simulink library "SUB_ECU_L4_MABX_HW_Interface"  (R2018a)
settings: Solver=VariableStepAuto  StartTime=0.0  StopTime=10.0  RelTol=1e-3
PostLoadFcn:
  | , if any(exist('dsrtsu_mdlpostloadfcn', 'file') == [2, 3, 6]), try dsrtsu_mdlpostloadfcn('Execute', bdroot); catch fprintf('Error in PostLoadFcn (dsrtsu_mdlpostloadfcn) for model "%s":\n %s\n', bdroot, lasterr); end, end,
undefined symbols (not defined in the file or in its folder): CANR_PROPB_REAX_3_13_CHANNEL_APV, CANR_PROPB_REAX_4_13_CHANNEL_APV, CANR_PROPB_XPR_1_50_CHANNEL_APV, ENUM_CAN_RX_T, ENUM_CAN_TX_T, ENUM_REAX_OPERATION_MODE_T, ENUM_SIGNAL_HEALTH_T, ENUM_XBR_CONTROL_MODE_T, ENUM_XBR_EBI_MODE_T, ENUM_XBR_PASS_THROUGH_ACTIVE_T, ENUM_XBR_PRIORITY_T, ENUM_XPR_INHIBIT_PARK_MANUAL_T, ENUM_XPR_INHIBIT_UNPARK_MANUAL_T, ENUM_XPR_PARK_MANUAL_T, ENUM_XPR_UNPARK_MANUAL_T, PROPB_REAX_1_E4_DES_POS_SIG_SRC_APV, PROPB_REAX_1_E4_DESIRED_OPMODE_APV, PROPB_REAX_1_E4_DESIRED_POSITION_APV, ptc_matlab_lib
libraries: PTC_MBDS_LIB x264, rtican x172, EmE_MBD_Blockset x39, simulink x34, $bdroot x16, rti1401lib_dio_type4 x8, simulink_need_slupdate x7, dsa_tcpip_lib x4, rti1401lib_adc_type4 x3, rtmapslib x3, rtitasklib x3
(part 14 of 51)

== system SUB_ECU_L4_MABX_HW_Interface/CAN_PIC_KW/CAN_RX_CCVS1_31/RX_CAN_31 ==
  Enable : Inport
  Bus Creator : BusCreator  Inputs=20
  Bus Creator3 : BusCreator  Inputs=4
  CCVS1_31 : rtican/RTICAN Receive (RX)   Reserved1=[]  Reserved2=[]  Reserved3=[]  Reserved4=[]  SfcnMessage=[]  Msg_Struct=[]  BoardTypeNo=[]  BoardNo=[]  ChannelNo=[]  Parameters=[]  DialogFcn=[]  UnitName=[]  Revision=[]  UnitValues=[]  DSProperties=struct('RTI',struct('Version',uint32(5),'BlockType',struct('isSLSource',uint8(1),'isSLSink',uint8(1),'isHWSource',uint8(0),'isHWSink',uint8(0),'isSetup',uint8(0),'isInline',uint8(1),'isNonInline',uint8(0),'isInterrupt',uint8(0),'isChannelwise',uint8(0)),'IOBoardType','RTICAN','UnitType','MESSAGE','Identifier','RX','DialogType','MSVC','BlockSet','RTICAN','SlaveProcessor','CAN'))  RTIBlockInterface=struct('OutputPortsWidth',int32([1 1 1 1 1 1 1 1 1 1 1 1 1 1 1 1 1 1 1 1 1 1 1]),'OutputPortsActive',ones(1,23),'OutputPortsName',{{'TwoSpeedAxleSwitch','ParkingBrakeSwitch','CruiseCtrlPauseSwitch','ParkBrakeReleaseInhibitRq','WheelBasedVehicleSpeed','CruiseCtrlActive','CruiseCtrlEnableSwitch','BrakeSwitch','ClutchSwitch','CruiseCtrlSetSwitch','CruiseCtrlCoastSwitch','CruiseCtrlResumeSwitch','CruiseCtrlAccelerateSwitch','CruiseCtrlSetSpeed','PTOGovernorState','CruiseCtrlStates','EngIdleIncrementSwitch','EngIdleDecrementSwitch','EngTestModeSwitch','EngShutdownOverrideSwitch',['RX status'],['RX time'],['RX delta time']}},'OutputPortsDataType',{{'SS_DOUBLE','SS_DOUBLE','SS_DOUBLE','SS_DOUBLE','SS_DOUBLE','SS_DOUBLE','SS_DOUBLE','SS_DOUBLE','SS_DOUBLE','SS_DOUBLE','SS_DOUBLE','SS_DOUBLE','SS_DOUBLE','SS_DOUBLE','SS_DOUBLE','SS_DOUBLE','SS_DOUBLE','SS_DOUBLE','SS_DOUBLE','SS_DOUBLE','SS_DOUBLE','SS_DOUBLE','SS_DOUBLE'}},'OutputPortsLabel',{{'TwoSpeedAxleSwitch','ParkingBrakeSwitch','CruiseCtrlPauseSwitch','ParkBrakeReleaseInhibitRq','WheelBasedVehicleSpeed','CruiseCtrlActive','CruiseCtrlEnableSwitch','BrakeSwitch','ClutchSwitch','CruiseCtrlSetSwitch','CruiseCtrlCoastSwitch','CruiseCtrlResumeSwitch','CruiseCtrlAccelerateSwitch','CruiseCtrlSetSpeed','PTOGovernorState','CruiseCtrlStates','EngIdleIncrementSwitch','EngIdleDecrementSwitch','EngTestModeSwitch','EngShutdownOverrideSwitch','','',''}},'OutputPortsLabelMode','ON','InputPortsWidth',int32(0),'InputPortsActive',0,'DialogFcn','rtican_message_interface_gui','BlockDisplay',{{'','center'}},'IconTransparency','on','ParameterTunableNames',{{}},'InitLevel',3,'BlockName',struct('Token',{{'CCVS1_31'}}),'SampleTime',{{-1}},'TriggerPort',{{'none'}},'EnablePort',{{'yes'}})  RTIBlockParameters=struct('BoardTypeNo',{{1,'OFF',[]}},'BoardNo',{{1,'ON',[1 16]}},'ChannelNo',{{1,'ON',[1 2]}},'Parameters',{{struct('DataFileSupport',struct('DataFileSelectedMaster',1,'DataFileSelectedLocal',0,'DataFileName','c:\localdata\chris\advanced_tech\adas\level4_rcp\truck1571\dbc\mabx_can1.dbc|','DataFileDate',{{{['03-Apr-2017 12:55:40']}}},'SelectedFile',['<no file selected>']),'Options',struct('StatusSelected',1,'TimeSelected',1,'DeltaTimeSelected',1,'BytePortSelected',0,'MessageLengthSelected',0,'TriggerPort',struct('Selected',0,'TriggerType',0),'UserCoding',struct('Selected',0,'InterfaceFile','UserDecodingFile','FcnName','UserDecodeFcn','InportSelected',0,'InportWidth',1,'OutportSelected',0,'OutportWidth',1),'EnablePortSelected',1,'SignalOnPortnameSelected',1,'UseRXService',1),'Message',struct('MsgOnBlocknameSelected',1,'MsgName','CCVS1_31','MsgIdFormat',1,'MsgId',419361073,'MsgLength',8,'NumSignals',20,'SampleTime',-1,'Signal',struct('SgnName',{'TwoSpeedAxleSwitch','ParkingBrakeSwitch','CruiseCtrlPauseSwitch','ParkBrakeReleaseInhibitRq','WheelBasedVehicleSpeed','CruiseCtrlActive','CruiseCtrlEnableSwitch','BrakeSwitch','ClutchSwitch','CruiseCtrlSetSwitch','CruiseCtrlCoastSwitch','CruiseCtrlResumeSwitch','CruiseCtrlAccelerateSwitch','CruiseCtrlSetSpeed','PTOGovernorState','CruiseCtrlStates','EngIdleIncrementSwitch','EngIdleDecrementSwitch','EngTestModeSwitch','EngShutdownOverrideSwitch'},'SgnStartBit',{0,2,4,6,8,24,26,28,30,32,34,36,38,40,48,53,56,58,60,62},'SgnLength',{2,2,2,2,16,2,2,2,2,2,2,2,2,8,5,3,2,2,2,2},'SgnType',{0,0,0,0,0,0,0,0,0,0,0,0,0,0,0,0,0,0,0,0},'ModeValue',{-1,-1,-1,-1,-1,-1,-1,-1,-1,-1,-1,-1,-1,-1,-1,-1,-1,-1,-1,-1},'DataType',{0,0,0,0,0,0,0,0,0,0,0,0,0,0,0,0,0,0,0,0},'ByteLayout',{0,0,0,0,0,0,0,0,0,0,0,0,0,0,0,0,0,0,0,0},'Factor',{1,1,1,1,2^-8,1,1,1,1,1,1,1,1,1,1,1,1,1,1,1},'Offset',{0,0,0,0,0,0,0,0,0,0,0,0,0,0,0,0,0,0,0,0},'SgnComment',{{['Switch signal which indicates the current axle range.']},{['Switch signal which indicates when the parking brake is set.']},{['Switch signal which indicates the position of the Cruise Control Pause Switch used on Remote Cruise Control applications.']},{['Park Brake Release Inhibit Request signals the desire that an applied park brake remain applied and limit the ability of the']},{['Speed of the vehicle as calculated from wheel or tailshaft speed.']},{['Cruise control is switched on.']},{['Switch signal which indicates that it is possible to manage the cruise control function.']},{['Switch signal which indicates that the driver operated brake foot pedal is being pressed.']},{['Switch signal which indicates that the clutch pedal is being pressed.']},{['Switch signal of the cruise control activator which indicates that the activator is in the position “set.']},{['Switch signal of the cruise control activator which indicates that the activator is in the position “coast (decelerate).']},{['Switch signal of the cruise control activator which indicates that the activator is in the position “resume.']},{['Switch signal of the cruise control activator which indicates that the activator is in the position “accelerate.']},{['Value of set (chosen) velocity of velocity control system.']},{['This parameter is used to indicate the current state or mode of operation by the power takeoff (PTO) governor.']},{['This parameter is used to indicate the current state, or mode, of operation by the cruise control device.']},{['Switch signal which indicates the position of the idle increment switch.']},{['Switch signal which indicates the position of the idle decrement switch.']},{['Switch signal which indicates the position of the engine test mode switch.']},{['Switch signal which indicates the position of the engine shutdown override switch.']}},'SgnUnit',{'','','','','km/h','','','','','','','','','km/h','','','','','',''},'Min',{0,0,0,0,0,0,0,0,0,0,0,0,0,0,0,0,0,0,0,0},'Max',{3,3,3,3,250.996,3,3,3,3,3,3,3,3,250,31,7,3,3,3,3},'SLDataType',{'SS_DOUBLE','SS_DOUBLE','SS_DOUBLE','SS_DOUBLE','SS_DOUBLE','SS_DOUBLE','SS_DOUBLE','SS_DOUBLE','SS_DOUBLE','SS_DOUBLE','SS_DOUBLE','SS_DOUBLE','SS_DOUBLE','SS_DOUBLE','SS_DOUBLE','SS_DOUBLE','SS_DOUBLE','SS_DOUBLE','SS_DOUBLE','SS_DOUBLE'}),'MsgIdNumFormat',1,'MsgComment',{{['Cruise Control/Vehicle Speed']}}),'Version',1.2,'general',struct('isFromLib',0)),'OFF',[]}},'GroupId',{{struct('Group',{{'RTICAN'}},'No',25,'Behavior',{{'NAMECHANGE'}},'BlockType',{{'SINK'}},'NameChangeFlag',0),'OFF',[]}},'SFcnRTICANMessage',{{struct('MsgType','RX','SFcnPortType','Scalar','MsgName','CCVS1_31','MsgIdFormat','XTD','MsgId',419361073,'MsgLength',8,'NumSignals',20,'SampleTime',-1,'Signal',struct('SgnName',{'TwoSpeedAxleSwitch','ParkingBrakeSwitch','CruiseCtrlPauseSwitch','ParkBrakeReleaseInhibitRq','WheelBasedVehicleSpeed','CruiseCtrlActive','CruiseCtrlEnableSwitch','BrakeSwitch','ClutchSwitch','CruiseCtrlSetSwitch','CruiseCtrlCoastSwitch','CruiseCtrlResumeSwitch','CruiseCtrlAccelerateSwitch','CruiseCtrlSetSpeed','PTOGovernorState','CruiseCtrlStates','EngIdleIncrementSwitch','EngIdleDecrementSwitch','EngTestModeSwitch','EngShutdownOverrideSwitch'},'SgnStartBit',{0,2,4,6,8,24,26,28,30,32,34,36,38,40,48,53,56,58,60,62},'SgnLength',{2,2,2,2,16,2,2,2,2,2,2,2,2,8,5,3,2,2,2,2},'SgnType',{'standard','standard','standard','standard','standard','standard','standard','standard','standard','standard','standard','standard','standard','standard','standard','standard','standard','standard','standard','standard'},'ModeValue',{-1,-1,-1,-1,-1,-1,-1,-1,-1,-1,-1,-1,-1,-1,-1,-1,-1,-1,-1,-1},'DataType',{['unsigned int'],['unsigned int'],['unsigned int'],['unsigned int'],['unsigned int'],['unsigned int'],['unsigned int'],['unsigned int'],['unsigned int'],['unsigned int'],['unsigned int'],['unsigned int'],['unsigned int'],['unsigned int'],['unsigned int'],['unsigned int'],['unsigned int'],['unsigned int'],['unsigned int'],['unsigned int']},'ByteLayout',{['little endian'],['little endian'],['little endian'],['little endian'],['little endian'],['little endian'],['little endian'],['little endian'],['little endian'],['little endian'],['little endian'],['little endian'],['little endian'],['little endian'],['little endian'],['little endian'],['little endian'],['little endian'],['little endian'],['little endian']},'Factor',{1,1,1,1,2^-8,1,1,1,1,1,1,1,1,1,1,1,1,1,1,1},'Offset',{0,0,0,0,0,0,0,0,0,0,0,0,0,0,0,0,0,0,0,0},'SLDataType',{'SS_DOUBLE','SS_DOUBLE','SS_DOUBLE','SS_DOUBLE','SS_DOUBLE','SS_DOUBLE','SS_DOUBLE','SS_DOUBLE','SS_DOUBLE','SS_DOUBLE','SS_DOUBLE','SS_DOUBLE','SS_DOUBLE','SS_DOUBLE','SS_DOUBLE','SS_DOUBLE','SS_DOUBLE','SS_DOUBLE','SS_DOUBLE','SS_DOUBLE'}),'StatusSelected','yes','TimeSelected','yes','DeltaTimeSelected','yes','BytePortSelected','no','MessageLengthSelected','no','TriggerPort',struct('Selected','no','TriggerType',0),'UserCoding',struct('Selected','no','InterfaceFile','UserDecodingFile','FcnName','UserDecodeFcn','InportSelected','no','InportWidth',1,'OutportSelected','no','OutportWidth',1),'EnablePortSelected','yes','UseRXService','yes','BoardType','DS1','BoardNo',1,'ControllerNo',1),'OFF',[]}},'TLCFileName',{{'rtican_rx_message','OFF',[]}})  RTISFcnParameters=struct('SFcnRTICANMessage','struct','TLCFileName','char')  RTIBlockParaDefault=struct('BoardTypeNo',4302,'BoardNo',1,'ChannelNo',1,'Parameters',struct('DataFileSupport',struct('DataFileSelectedMaster',0,'DataFileSelectedLocal',0,'DataFileName','','DataFileDate','','SelectedFile',['<no file selected>']),'Options',struct('StatusSelected',1,'TimeSelected',1,'DeltaTimeSelected',1,'BytePortSelected',0,'MessageLengthSelected',0,'TriggerPort',struct('Selected',0,'TriggerType','rising'),'UserCoding',struct('Selected',0,'InterfaceFile','UserDecodingFile','FcnName','UserDecodeFcn','InportSelected',0,'InportWidth',1,'OutportSelected',0,'OutportWidth',1),'EnablePortSelected',0,'SignalOnPortnameSelected',1,'UseRXService',0),'Message',struct('MsgOnBlocknameSelected',0,'MsgName',['RX Message'],'MsgIdFormat',0,'MsgId',100,'MsgLength',8,'NumSignals',1,'SampleTime',-1,'Signal',struct('SgnName',['RX signal'],'SgnStartBit',0,'SgnLength',8,'SgnType',0,'ModeValue',-1,'DataType',0,'SLDataType','SS_DOUBLE','ByteLayout',0,'Factor',1,'Offset',0,'Min',0,'Max',255,'SgnComment',{{}},'SgnUnit',''),'MsgIdNumFormat',0,'MsgComment',{{''}}),'Version',1.2,'general',struct('isFromLib',1)),'GroupId',struct('Group',{{'RTICAN'}},'No',1,'Behavior',{{'NAMECHANGE'}},'BlockType',{{'SINK'}},'NameChangeFlag',0),'SFcnRTICANMessage',struct('MsgType','RX','MsgName',['RX Message'],'MsgIdFormat','STD','MsgId',100,'MsgLength',8,'NumSignals',1,'SampleTime',-1,'Signal',struct('SgnName',['RX signal'],'SgnStartBit',0,'SgnLength',8,'SgnType','standard','ModeValue',-1,'DataType',['unsigned int'],'ByteLayout',['little endian'],'SLDataType','SS_DOUBLE','Factor',1,'Offset',0),'StatusSelected','yes','TimeSelected','yes','DeltaTimeSelected','yes','BytePortSelected','no','MessageLengthSelected','no','EnablePortSelected','no','UserCoding',struct('Selected','no','InterfaceFile','UserDecodingFile','FcnName','UserDecodeFcn','InportSelected','no','InportWidth',1,'OutportSelected','no','OutportWidth',1),'TriggerPort',struct('Selected','no','TriggerType','rising'),'UseRXService','no','BoardType','DS4302','BoardNo',1,'ControllerNo',1,'SFcnPortType','Scalar'),'TLCFileName','rtican_rx_message')
      settings: AttributesFormatString=Group Id: RTICAN25\n  SourceProductName=dSPACE RTI CAN Blockset
  Data Type Conversion10 : DataTypeConversion  OutDataTypeStr=double  SaturateOnIntegerOverflow=on
  Data Type Conversion8 : DataTypeConversion  OutDataTypeStr=boolean  SaturateOnIntegerOverflow=on
  Data Type Conversion9 : DataTypeConversion  OutDataTypeStr=double  SaturateOnIntegerOverflow=on
  CCVS1_31_ : Outport
  wires:
  Bus Creator3/1 -> CCVS1_31_/1  "CCVS1_31"
  Bus Creator/1 -> Bus Creator3/1  "CCVS31Data"
  Enable/1 -> CCVS1_31/Enable
  CCVS1_31/23 -> Data Type Conversion10/1
  CCVS1_31/22 -> Data Type Conversion9/1
  CCVS1_31/21 -> Data Type Conversion8/1
  Data Type Conversion8/1 -> Bus Creator3/2  "RX_status"
  Data Type Conversion10/1 -> Bus Creator3/4  "RX_delta_time"
  Data Type Conversion9/1 -> Bus Creator3/3  "RX_time"
  CCVS1_31/13 -> Bus Creator/13  "CruiseCtrlAccelerateSwitch"
  CCVS1_31/12 -> Bus Creator/12  "CruiseCtrlResumeSwitch"
  CCVS1_31/11 -> Bus Creator/11  "CruiseCtrlCoastSwitch"
  CCVS1_31/16 -> Bus Creator/16  "CruiseCtrlStates"
  CCVS1_31/14 -> Bus Creator/14  "CruiseCtrlSetSpeed"
  CCVS1_31/15 -> Bus Creator/15  "PTOGovernorState"
  CCVS1_31/8 -> Bus Creator/8  "BrakeSwitch"
  CCVS1_31/9 -> Bus Creator/9  "ClutchSwitch"
  CCVS1_31/10 -> Bus Creator/10  "CruiseCtrlSetSwitch"
  CCVS1_31/7 -> Bus Creator/7  "CruiseCtrlEnableSwitch"
  CCVS1_31/20 -> Bus Creator/20  "EngShutdownOverrideSwitch"
  CCVS1_31/19 -> Bus Creator/19  "EngTestModeSwitch"
  CCVS1_31/18 -> Bus Creator/18  "EngIdleDecrementSwitch"
  CCVS1_31/17 -> Bus Creator/17  "EngIdleIncrementSwitch"
  CCVS1_31/2 -> Bus Creator/2  "ParkingBrakeSwitch"
  CCVS1_31/1 -> Bus Creator/1  "TwoSpeedAxleSwitch"
  CCVS1_31/3 -> Bus Creator/3  "CruiseCtrlPauseSwitch"
  CCVS1_31/4 -> Bus Creator/4  "ParkBrakeReleaseInhibitRq"
  CCVS1_31/6 -> Bus Creator/6  "CruiseCtrlActive"
  CCVS1_31/5 -> Bus Creator/5  "WheelBasedVehicleSpeed"

== system SUB_ECU_L4_MABX_HW_Interface/CAN_PIC_KW/CAN_RX_COGSOGRapidUpdate_01/RX_CAN_4 ==
  Enable : Inport
  Bus Creator1 : BusCreator  Inputs=7
  Bus Creator3 : BusCreator  Inputs=7
  COGSOGRapidUpdate_00 : rtican/RTICAN Receive (RX)   Reserved1=[]  Reserved2=[]  Reserved3=[]  Reserved4=[]  SfcnMessage=[]  Msg_Struct=[]  BoardTypeNo=[]  BoardNo=[]  ChannelNo=[]  Parameters=[]  DialogFcn=[]  UnitName=[]  Revision=[]  UnitValues=[]  DSProperties=struct('RTI',struct('Version',uint32(5),'BlockType',struct('isSLSource',uint8(1),'isSLSink',uint8(1),'isHWSource',uint8(0),'isHWSink',uint8(0),'isSetup',uint8(0),'isInline',uint8(1),'isNonInline',uint8(0),'isInterrupt',uint8(0),'isChannelwise',uint8(0)),'IOBoardType','RTICAN','UnitType','MESSAGE','Identifier','RX','DialogType','MSVC','BlockSet','RTICAN','SlaveProcessor','CAN'))  RTIBlockInterface=struct('OutputPortsWidth',int32([1 1 1 1 1 1 1]),'OutputPortsActive',[1 1 1 1 1 1 1],'OutputPortsName',{{'SID','COGReference','CourseOverGround','SpeedOverGround',['RX status'],['RX time'],['RX delta time']}},'OutputPortsDataType',{{'SS_DOUBLE','SS_DOUBLE','SS_DOUBLE','SS_DOUBLE','SS_DOUBLE','SS_DOUBLE','SS_DOUBLE'}},'OutputPortsLabel',{{'SID','COGReference','CourseOverGround','SpeedOverGround','','',''}},'OutputPortsLabelMode','ON','InputPortsWidth',int32(0),'InputPortsActive',0,'DialogFcn','rtican_message_interface_gui','BlockDisplay',{{'','center'}},'IconTransparency','on','ParameterTunableNames',{{}},'InitLevel',3,'BlockName',struct('Token',{{'COGSOGRapidUpdate_00'}}),'SampleTime',{{-1}},'TriggerPort',{{'none'}},'EnablePort',{{'yes'}})  RTIBlockParameters=struct('BoardTypeNo',{{1,'OFF',[]}},'BoardNo',{{2,'ON',[1 16]}},'ChannelNo',{{2,'ON',[1 2]}},'Parameters',{{struct('DataFileSupport',struct('DataFileSelectedMaster',1,'DataFileSelectedLocal',0,'DataFileName','c:\localdata\chris\advanced_tech\adas\level4_rcp\truck1571\dbc\mabx_can4.dbc|','DataFileDate',{{{['10-Feb-2017 15:17:28']}}},'SelectedFile',['<no file selected>']),'Options',struct('StatusSelected',1,'TimeSelected',1,'DeltaTimeSelected',1,'BytePortSelected',0,'MessageLengthSelected',0,'TriggerPort',struct('Selected',0,'TriggerType',0),'UserCoding',struct('Selected',0,'InterfaceFile','UserDecodingFile','FcnName','UserDecodeFcn','InportSelected',0,'InportWidth',1,'OutportSelected',0,'OutportWidth',1),'EnablePortSelected',1,'SignalOnPortnameSelected',1,'UseRXService',1),'Message',struct('MsgOnBlocknameSelected',1,'MsgName','COGSOGRapidUpdate_00','MsgIdFormat',1,'MsgId',167248384,'MsgLength',8,'NumSignals',4,'SampleTime',-1,'Signal',struct('SgnName',{'SID','COGReference','CourseOverGround','SpeedOverGround'},'SgnStartBit',{0,8,16,32},'SgnLength',{8,2,16,16},'SgnType',{0,0,0,0},'ModeValue',{-1,-1,-1,-1},'DataType',{0,0,0,0},'ByteLayout',{0,0,0,0},'Factor',{1,1,0.0001,0.01},'Offset',{0,0,0,0},'SgnComment',{{['An upward counting number used to tie related information together between different PGNs.For example,SID would be used to tie together COG,SOG and RAIM values to a given Pos.255=no valid Pos fix to tie it to.Range 0 to 250 for valid Pos fixes.']},{['0 = True, ' char(10) '1 = Magnetic, ' char(10) '2 = Error, ' char(10) '3 = Null']},{['The direction of the path over ground actually followed by a vessel.']},{''}},'SgnUnit',{'','','rad','m/s'},'Min',{0,0,0,0},'Max',{252,3,6.28318,655.32},'SLDataType',{'SS_DOUBLE','SS_DOUBLE','SS_DOUBLE','SS_DOUBLE'}),'MsgIdNumFormat',1,'MsgComment',{{['This PGN is a single frame PGN that provides Course Over Ground(COG)and Speed Over Ground(SOG).' char(10) '' char(10) 'Being a ']}}),'Version',1.2,'general',struct('isFromLib',0)),'OFF',[]}},'GroupId',{{struct('Group',{{'RTICAN'}},'No',28,'Behavior',{{'NAMECHANGE'}},'BlockType',{{'SINK'}},'NameChangeFlag',0),'OFF',[]}},'SFcnRTICANMessage',{{struct('MsgType','RX','SFcnPortType','Scalar','MsgName','COGSOGRapidUpdate_00','MsgIdFormat','XTD','MsgId',167248384,'MsgLength',8,'NumSignals',4,'SampleTime',-1,'Signal',struct('SgnName',{'SID','COGReference','CourseOverGround','SpeedOverGround'},'SgnStartBit',{0,8,16,32},'SgnLength',{8,2,16,16},'SgnType',{'standard','standard','standard','standard'},'ModeValue',{-1,-1,-1,-1},'DataType',{['unsigned int'],['unsigned int'],['unsigned int'],['unsigned int']},'ByteLayout',{['little endian'],['little endian'],['little endian'],['little endian']},'Factor',{1,1,0.0001,0.01},'Offset',{0,0,0,0},'SLDataType',{'SS_DOUBLE','SS_DOUBLE','SS_DOUBLE','SS_DOUBLE'}),'StatusSelected','yes','TimeSelected','yes','DeltaTimeSelected','yes','BytePortSelected','no','MessageLengthSelected','no','TriggerPort',struct('Selected','no','TriggerType',0),'UserCoding',struct('Selected','no','InterfaceFile','UserDecodingFile','FcnName','UserDecodeFcn','InportSelected','no','InportWidth',1,'OutportSelected','no','OutportWidth',1),'EnablePortSelected','yes','UseRXService','yes','BoardType','DS1','BoardNo',2,'ControllerNo',2),'OFF',[]}},'TLCFileName',{{'rtican_rx_message','OFF',[]}})  RTISFcnParameters=struct('SFcnRTICANMessage','struct','TLCFileName','char')  RTIBlockParaDefault=struct('BoardTypeNo',4302,'BoardNo',1,'ChannelNo',1,'Parameters',struct('DataFileSupport',struct('DataFileSelectedMaster',0,'DataFileSelectedLocal',0,'DataFileName','','DataFileDate','','SelectedFile',['<no file selected>']),'Options',struct('StatusSelected',1,'TimeSelected',1,'DeltaTimeSelected',1,'BytePortSelected',0,'MessageLengthSelected',0,'TriggerPort',struct('Selected',0,'TriggerType','rising'),'UserCoding',struct('Selected',0,'InterfaceFile','UserDecodingFile','FcnName','UserDecodeFcn','InportSelected',0,'InportWidth',1,'OutportSelected',0,'OutportWidth',1),'EnablePortSelected',0,'SignalOnPortnameSelected',1,'UseRXService',0),'Message',struct('MsgOnBlocknameSelected',0,'MsgName',['RX Message'],'MsgIdFormat',0,'MsgId',100,'MsgLength',8,'NumSignals',1,'SampleTime',-1,'Signal',struct('SgnName',['RX signal'],'SgnStartBit',0,'SgnLength',8,'SgnType',0,'ModeValue',-1,'DataType',0,'SLDataType','SS_DOUBLE','ByteLayout',0,'Factor',1,'Offset',0,'Min',0,'Max',255,'SgnComment',{{}},'SgnUnit',''),'MsgIdNumFormat',0,'MsgComment',{{''}}),'Version',1.2,'general',struct('isFromLib',1)),'GroupId',struct('Group',{{'RTICAN'}},'No',1,'Behavior',{{'NAMECHANGE'}},'BlockType',{{'SINK'}},'NameChangeFlag',0),'SFcnRTICANMessage',struct('MsgType','RX','MsgName',['RX Message'],'MsgIdFormat','STD','MsgId',100,'MsgLength',8,'NumSignals',1,'SampleTime',-1,'Signal',struct('SgnName',['RX signal'],'SgnStartBit',0,'SgnLength',8,'SgnType','standard','ModeValue',-1,'DataType',['unsigned int'],'ByteLayout',['little endian'],'SLDataType','SS_DOUBLE','Factor',1,'Offset',0),'StatusSelected','yes','TimeSelected','yes','DeltaTimeSelected','yes','BytePortSelected','no','MessageLengthSelected','no','EnablePortSelected','no','UserCoding',struct('Selected','no','InterfaceFile','UserDecodingFile','FcnName','UserDecodeFcn','InportSelected','no','InportWidth',1,'OutportSelected','no','OutportWidth',1),'TriggerPort',struct('Selected','no','TriggerType','rising'),'UseRXService','no','BoardType','DS4302','BoardNo',1,'ControllerNo',1,'SFcnPortType','Scalar'),'TLCFileName','rtican_rx_message')
      settings: AttributesFormatString=Group Id: RTICAN28\n  SourceProductName=dSPACE RTI CAN Blockset
  COGSOGRapidUpdate_1 : rtican/RTICAN Receive (RX)   Reserved1=[]  Reserved2=[]  Reserved3=[]  Reserved4=[]  SfcnMessage=[]  Msg_Struct=[]  BoardTypeNo=[]  BoardNo=[]  ChannelNo=[]  Parameters=[]  DialogFcn=[]  UnitName=[]  Revision=[]  UnitValues=[]  DSProperties=struct('RTI',struct('Version',uint32(5),'BlockType',struct('isSLSource',uint8(1),'isSLSink',uint8(1),'isHWSource',uint8(0),'isHWSink',uint8(0),'isSetup',uint8(0),'isInline',uint8(1),'isNonInline',uint8(0),'isInterrupt',uint8(0),'isChannelwise',uint8(0)),'IOBoardType','RTICAN','UnitType','MESSAGE','Identifier','RX','DialogType','MSVC','BlockSet','RTICAN','SlaveProcessor','CAN'))  RTIBlockInterface=struct('OutputPortsWidth',int32([1 1 1 1 1 1 1]),'OutputPortsActive',[1 1 1 1 1 1 1],'OutputPortsName',{{'SID','COGReference','CourseOverGround','SpeedOverGround',['RX status'],['RX time'],['RX delta time']}},'OutputPortsDataType',{{'SS_DOUBLE','SS_DOUBLE','SS_DOUBLE','SS_DOUBLE','SS_DOUBLE','SS_DOUBLE','SS_DOUBLE'}},'OutputPortsLabel',{{'SID','COGReference','CourseOverGround','SpeedOverGround','','',''}},'OutputPortsLabelMode','ON','InputPortsWidth',int32(0),'InputPortsActive',0,'DialogFcn','rtican_message_interface_gui','BlockDisplay',{{'','center'}},'IconTransparency','on','ParameterTunableNames',{{}},'InitLevel',3,'BlockName',struct('Token',{{'COGSOGRapidUpdate_00'}}),'SampleTime',{{-1}},'TriggerPort',{{'none'}},'EnablePort',{{'yes'}})  RTIBlockParameters=struct('BoardTypeNo',{{1,'OFF',[]}},'BoardNo',{{2,'ON',[1 16]}},'ChannelNo',{{2,'ON',[1 2]}},'Parameters',{{struct('DataFileSupport',struct('DataFileSelectedMaster',1,'DataFileSelectedLocal',0,'DataFileName',['c:\localdata\chris\advanced_tech\adas\ptc_autonomous_truck_secure\branches\truck1571\dbc\mabx_can4.dbc|c:\localdata\chris\advanced_tech\adas\ptc_autonomous_truck_secure\branches\svn\powertrainsys\trunk\src\projects_rcp\my2017_rcp\dbc files\j1939.dbc|'],'DataFileDate',{{{['10-Feb-2017 15:17:28']}}},'SelectedFile',['<no file selected>']),'Options',struct('StatusSelected',1,'TimeSelected',1,'DeltaTimeSelected',1,'BytePortSelected',0,'MessageLengthSelected',0,'TriggerPort',struct('Selected',0,'TriggerType',0),'UserCoding',struct('Selected',0,'InterfaceFile','UserDecodingFile','FcnName','UserDecodeFcn','InportSelected',0,'InportWidth',1,'OutportSelected',0,'OutportWidth',1),'EnablePortSelected',1,'SignalOnPortnameSelected',1,'UseRXService',1),'Message',struct('MsgOnBlocknameSelected',1,'MsgName','COGSOGRapidUpdate_00','MsgIdFormat',1,'MsgId',167248385,'MsgLength',8,'NumSignals',4,'SampleTime',-1,'Signal',struct('SgnName',{'SID','COGReference','CourseOverGround','SpeedOverGround'},'SgnStartBit',{0,8,16,32},'SgnLength',{8,2,16,16},'SgnType',{0,0,0,0},'ModeValue',{-1,-1,-1,-1},'DataType',{0,0,0,0},'ByteLayout',{0,0,0,0},'Factor',{1,1,0.0001,0.01},'Offset',{0,0,0,0},'SgnComment',{{['An upward counting number used to tie related information together between different PGNs.For example,SID would be used to tie together COG,SOG and RAIM values to a given Pos.255=no valid Pos fix to tie it to.Range 0 to 250 for valid Pos fixes.']},{['0 = True, ' char(10) '1 = Magnetic, ' char(10) '2 = Error, ' char(10) '3 = Null']},{['The direction of the path over ground actually followed by a vessel.']},{''}},'SgnUnit',{'','','rad','m/s'},'Min',{0,0,0,0},'Max',{252,3,6.28318,655.32},'SLDataType',{'SS_DOUBLE','SS_DOUBLE','SS_DOUBLE','SS_DOUBLE'}),'MsgIdNumFormat',1,'MsgComment',{{['This PGN is a single frame PGN that provides Course Over Ground(COG)and Speed Over Ground(SOG).' char(10) '' char(10) 'Being a ']}}),'Version',1.2,'general',struct('isFromLib',0)),'OFF',[]}},'GroupId',{{struct('Group',{{'RTICAN'}},'No',28,'Behavior',{{'NAMECHANGE'}},'BlockType',{{'SINK'}},'NameChangeFlag',0),'OFF',[]}},'SFcnRTICANMessage',{{struct('MsgType','RX','SFcnPortType','Scalar','MsgName','COGSOGRapidUpdate_00','MsgIdFormat','XTD','MsgId',167248385,'MsgLength',8,'NumSignals',4,'SampleTime',-1,'Signal',struct('SgnName',{'SID','COGReference','CourseOverGround','SpeedOverGround'},'SgnStartBit',{0,8,16,32},'SgnLength',{8,2,16,16},'SgnType',{'standard','standard','standard','standard'},'ModeValue',{-1,-1,-1,-1},'DataType',{['unsigned int'],['unsigned int'],['unsigned int'],['unsigned int']},'ByteLayout',{['little endian'],['little endian'],['little endian'],['little endian']},'Factor',{1,1,0.0001,0.01},'Offset',{0,0,0,0},'SLDataType',{'SS_DOUBLE','SS_DOUBLE','SS_DOUBLE','SS_DOUBLE'}),'StatusSelected','yes','TimeSelected','yes','DeltaTimeSelected','yes','BytePortSelected','no','MessageLengthSelected','no','TriggerPort',struct('Selected','no','TriggerType',0),'UserCoding',struct('Selected','no','InterfaceFile','UserDecodingFile','FcnName','UserDecodeFcn','InportSelected','no','InportWidth',1,'OutportSelected','no','OutportWidth',1),'EnablePortSelected','yes','UseRXService','yes','BoardType','DS1','BoardNo',2,'ControllerNo',2),'OFF',[]}},'TLCFileName',{{'rtican_rx_message','OFF',[]}})  RTISFcnParameters=struct('SFcnRTICANMessage','struct','TLCFileName','char')  RTIBlockParaDefault=struct('BoardTypeNo',4302,'BoardNo',1,'ChannelNo',1,'Parameters',struct('DataFileSupport',struct('DataFileSelectedMaster',0,'DataFileSelectedLocal',0,'DataFileName','','DataFileDate','','SelectedFile',['<no file selected>']),'Options',struct('StatusSelected',1,'TimeSelected',1,'DeltaTimeSelected',1,'BytePortSelected',0,'MessageLengthSelected',0,'TriggerPort',struct('Selected',0,'TriggerType','rising'),'UserCoding',struct('Selected',0,'InterfaceFile','UserDecodingFile','FcnName','UserDecodeFcn','InportSelected',0,'InportWidth',1,'OutportSelected',0,'OutportWidth',1),'EnablePortSelected',0,'SignalOnPortnameSelected',1,'UseRXService',0),'Message',struct('MsgOnBlocknameSelected',0,'MsgName',['RX Message'],'MsgIdFormat',0,'MsgId',100,'MsgLength',8,'NumSignals',1,'SampleTime',-1,'Signal',struct('SgnName',['RX signal'],'SgnStartBit',0,'SgnLength',8,'SgnType',0,'ModeValue',-1,'DataType',0,'SLDataType','SS_DOUBLE','ByteLayout',0,'Factor',1,'Offset',0,'Min',0,'Max',255,'SgnComment',{{}},'SgnUnit',''),'MsgIdNumFormat',0,'MsgComment',{{''}}),'Version',1.2,'general',struct('isFromLib',1)),'GroupId',struct('Group',{{'RTICAN'}},'No',1,'Behavior',{{'NAMECHANGE'}},'BlockType',{{'SINK'}},'NameChangeFlag',0),'SFcnRTICANMessage',struct('MsgType','RX','MsgName',['RX Message'],'MsgIdFormat','STD','MsgId',100,'MsgLength',8,'NumSignals',1,'SampleTime',-1,'Signal',struct('SgnName',['RX signal'],'SgnStartBit',0,'SgnLength',8,'SgnType','standard','ModeValue',-1,'DataType',['unsigned int'],'ByteLayout',['little endian'],'SLDataType','SS_DOUBLE','Factor',1,'Offset',0),'StatusSelected','yes','TimeSelected','yes','DeltaTimeSelected','yes','BytePortSelected','no','MessageLengthSelected','no','EnablePortSelected','no','UserCoding',struct('Selected','no','InterfaceFile','UserDecodingFile','FcnName','UserDecodeFcn','InportSelected','no','InportWidth',1,'OutportSelected','no','OutportWidth',1),'TriggerPort',struct('Selected','no','TriggerType','rising'),'UseRXService','no','BoardType','DS4302','BoardNo',1,'ControllerNo',1,'SFcnPortType','Scalar'),'TLCFileName','rtican_rx_message')
      settings: AttributesFormatString=Group Id: RTICAN28\n  SourceProductName=dSPACE RTI CAN Blockset
  Data Type Conversion1 : DataTypeConversion  OutDataTypeStr=boolean  SaturateOnIntegerOverflow=on
  Data Type Conversion{2..3,9..10} (4 alike) : DataTypeConversion  OutDataTypeStr=double  SaturateOnIntegerOverflow=on
  Data Type Conversion8 : DataTypeConversion  OutDataTypeStr=boolean  SaturateOnIntegerOverflow=on
  Switch : Switch  Criteria=u2 ~= 0
  COGSOGRapidUpdate_01 : Outport
  wires:
  COGSOGRapidUpdate_00/1 -> Bus Creator3/1  "SID"
  COGSOGRapidUpdate_00/2 -> Bus Creator3/2  "COGReference"
  COGSOGRapidUpdate_00/3 -> Bus Creator3/3  "CourseOverGround"
  COGSOGRapidUpdate_00/4 -> Bus Creator3/4  "SpeedOverGround"
  Bus Creator3/1 -> Switch/1  "COGSOGRapidUpdate_01"
  Enable/1 -> COGSOGRapidUpdate_1/Enable, COGSOGRapidUpdate_00/Enable
  COGSOGRapidUpdate_00/7 -> Data Type Conversion10/1
  COGSOGRapidUpdate_00/6 -> Data Type Conversion9/1
  COGSOGRapidUpdate_00/5 -> Data Type Conversion8/1
  Data Type Conversion8/1 -> Switch/2, Bus Creator3/5  "RX_status"
  Data Type Conversion10/1 -> Bus Creator3/7  "RX_delta_time"
  Data Type Conversion9/1 -> Bus Creator3/6  "RX_time"
  COGSOGRapidUpdate_1/1 -> Bus Creator1/1  "SID"
  COGSOGRapidUpdate_1/2 -> Bus Creator1/2  "COGReference"
  COGSOGRapidUpdate_1/3 -> Bus Creator1/3  "CourseOverGround"
  COGSOGRapidUpdate_1/4 -> Bus Creator1/4  "SpeedOverGround"
  COGSOGRapidUpdate_1/5 -> Data Type Conversion1/1
  COGSOGRapidUpdate_1/6 -> Data Type Conversion2/1
  COGSOGRapidUpdate_1/7 -> Data Type Conversion3/1
  Data Type Conversion1/1 -> Bus Creator1/5  "RX_status"
  Data Type Conversion2/1 -> Bus Creator1/6  "RX_time"
  Data Type Conversion3/1 -> Bus Creator1/7  "RX_delta_time"
  Switch/1 -> COGSOGRapidUpdate_01/1
  Bus Creator1/1 -> Switch/3

== system SUB_ECU_L4_MABX_HW_Interface/CAN_PIC_KW/CAN_RX_CVW_0B/RX_CAN_1 ==
  Enable : Inport
  Bus Creator3 : BusCreator  Inputs=4
  CVW_0B1 : rtican/RTICAN Receive (RX)   Reserved1=[]  Reserved2=[]  Reserved3=[]  Reserved4=[]  SfcnMessage=[]  Msg_Struct=[]  BoardTypeNo=[]  BoardNo=[]  ChannelNo=[]  Parameters=[]  DialogFcn=[]  UnitName=[]  Revision=[]  UnitValues=[]  DSProperties=struct('RTI',struct('Version',uint32(5),'BlockType',struct('isSLSource',uint8(1),'isSLSink',uint8(1),'isHWSource',uint8(0),'isHWSink',uint8(0),'isSetup',uint8(0),'isInline',uint8(1),'isNonInline',uint8(0),'isInterrupt',uint8(0),'isChannelwise',uint8(0)),'IOBoardType','RTICAN','UnitType','MESSAGE','Identifier','RX','DialogType','MSVC','BlockSet','RTICAN','SlaveProcessor','CAN'))  RTIBlockInterface=struct('OutputPortsWidth',int32([1 1 1 1]),'OutputPortsActive',[1 1 1 1],'OutputPortsName',{{'SPN1760_GrossCombinationVehicleWeight',['RX status'],['RX time'],['RX delta time']}},'OutputPortsDataType',{{'SS_DOUBLE','SS_DOUBLE','SS_DOUBLE','SS_DOUBLE'}},'OutputPortsLabel',{{'SPN1760_GrossCombinationVehicleWeight','','',''}},'OutputPortsLabelMode','ON','InputPortsWidth',int32(0),'InputPortsActive',0,'DialogFcn','rtican_message_interface_gui','BlockDisplay',{{'','center'}},'IconTransparency','on','ParameterTunableNames',{{}},'InitLevel',3,'BlockName',struct('Token',{{'CVW_0B'}}),'SampleTime',{{-1}},'TriggerPort',{{'none'}},'EnablePort',{{'yes'}})  RTIBlockParameters=struct('BoardTypeNo',{{1,'OFF',[]}},'BoardNo',{{1,'ON',[1 16]}},'ChannelNo',{{1,'ON',[1 2]}},'Parameters',{{struct('DataFileSupport',struct('DataFileSelectedMaster',1,'DataFileSelectedLocal',0,'DataFileName','i:\435\team\balton\truck1571\dbc\mabx_can1.dbc|','DataFileDate',{{{['03-Apr-2017 12:55:40']}}},'SelectedFile',['<no file selected>']),'Options',struct('StatusSelected',1,'TimeSelected',1,'DeltaTimeSelected',1,'BytePortSelected',0,'MessageLengthSelected',0,'TriggerPort',struct('Selected',0,'TriggerType',0),'UserCoding',struct('Selected',0,'InterfaceFile','UserDecodingFile','FcnName','UserDecodeFcn','InportSelected',0,'InportWidth',1,'OutportSelected',0,'OutportWidth',1),'EnablePortSelected',1,'SignalOnPortnameSelected',1,'UseRXService',1),'Message',struct('MsgOnBlocknameSelected',1,'MsgName','CVW_0B','MsgIdFormat',1,'MsgId',419328011,'MsgLength',8,'NumSignals',1,'SampleTime',-1,'Signal',struct('SgnName','SPN1760_GrossCombinationVehicleWeight','SgnStartBit',16,'SgnLength',16,'SgnType',0,'ModeValue',-1,'DataType',0,'ByteLayout',0,'Factor',10,'Offset',0,'SgnComment',{{['Switch signal which indicates when the parking brake is set.']}},'SgnUnit','kg','Min',0,'Max',3,'SLDataType','SS_DOUBLE'),'MsgIdNumFormat',1,'MsgComment',{{['Combination Vehicle Weight']}}),'Version',1.2,'general',struct('isFromLib',0)),'OFF',[]}},'GroupId',{{struct('Group',{{'RTICAN'}},'No',25,'Behavior',{{'NAMECHANGE'}},'BlockType',{{'SINK'}},'NameChangeFlag',0),'OFF',[]}},'SFcnRTICANMessage',{{struct('MsgType','RX','SFcnPortType','Scalar','MsgName','CVW_0B','MsgIdFormat','XTD','MsgId',419328011,'MsgLength',8,'NumSignals',1,'SampleTime',-1,'Signal',struct('SgnName','SPN1760_GrossCombinationVehicleWeight','SgnStartBit',16,'SgnLength',16,'SgnType','standard','ModeValue',-1,'DataType',['unsigned int'],'ByteLayout',['little endian'],'Factor',10,'Offset',0,'SLDataType','SS_DOUBLE'),'StatusSelected','yes','TimeSelected','yes','DeltaTimeSelected','yes','BytePortSelected','no','MessageLengthSelected','no','TriggerPort',struct('Selected','no','TriggerType',0),'UserCoding',struct('Selected','no','InterfaceFile','UserDecodingFile','FcnName','UserDecodeFcn','InportSelected','no','InportWidth',1,'OutportSelected','no','OutportWidth',1),'EnablePortSelected','yes','UseRXService','yes','BoardType','DS1','BoardNo',1,'ControllerNo',1),'OFF',[]}},'TLCFileName',{{'rtican_rx_message','OFF',[]}})  RTISFcnParameters=struct('SFcnRTICANMessage','struct','TLCFileName','char')  RTIBlockParaDefault=struct('BoardTypeNo',4302,'BoardNo',1,'ChannelNo',1,'Parameters',struct('DataFileSupport',struct('DataFileSelectedMaster',0,'DataFileSelectedLocal',0,'DataFileName','','DataFileDate','','SelectedFile',['<no file selected>']),'Options',struct('StatusSelected',1,'TimeSelected',1,'DeltaTimeSelected',1,'BytePortSelected',0,'MessageLengthSelected',0,'TriggerPort',struct('Selected',0,'TriggerType','rising'),'UserCoding',struct('Selected',0,'InterfaceFile','UserDecodingFile','FcnName','UserDecodeFcn','InportSelected',0,'InportWidth',1,'OutportSelected',0,'OutportWidth',1),'EnablePortSelected',0,'SignalOnPortnameSelected',1,'UseRXService',0),'Message',struct('MsgOnBlocknameSelected',0,'MsgName',['RX Message'],'MsgIdFormat',0,'MsgId',100,'MsgLength',8,'NumSignals',1,'SampleTime',-1,'Signal',struct('SgnName',['RX signal'],'SgnStartBit',0,'SgnLength',8,'SgnType',0,'ModeValue',-1,'DataType',0,'SLDataType','SS_DOUBLE','ByteLayout',0,'Factor',1,'Offset',0,'Min',0,'Max',255,'SgnComment',{{}},'SgnUnit',''),'MsgIdNumFormat',0,'MsgComment',{{''}}),'Version',1.2,'general',struct('isFromLib',1)),'GroupId',struct('Group',{{'RTICAN'}},'No',1,'Behavior',{{'NAMECHANGE'}},'BlockType',{{'SINK'}},'NameChangeFlag',0),'SFcnRTICANMessage',struct('MsgType','RX','MsgName',['RX Message'],'MsgIdFormat','STD','MsgId',100,'MsgLength',8,'NumSignals',1,'SampleTime',-1,'Signal',struct('SgnName',['RX signal'],'SgnStartBit',0,'SgnLength',8,'SgnType','standard','ModeValue',-1,'DataType',['unsigned int'],'ByteLayout',['little endian'],'SLDataType','SS_DOUBLE','Factor',1,'Offset',0),'StatusSelected','yes','TimeSelected','yes','DeltaTimeSelected','yes','BytePortSelected','no','MessageLengthSelected','no','EnablePortSelected','no','UserCoding',struct('Selected','no','InterfaceFile','UserDecodingFile','FcnName','UserDecodeFcn','InportSelected','no','InportWidth',1,'OutportSelected','no','OutportWidth',1),'TriggerPort',struct('Selected','no','TriggerType','rising'),'UseRXService','no','BoardType','DS4302','BoardNo',1,'ControllerNo',1,'SFcnPortType','Scalar'),'TLCFileName','rtican_rx_message')
      settings: AttributesFormatString=Group Id: RTICAN25\n  SourceProductName=dSPACE RTI CAN Blockset
  Data Type Conversion1 : DataTypeConversion  OutDataTypeStr=double  SaturateOnIntegerOverflow=on
  Data Type Conversion10 : DataTypeConversion  OutDataTypeStr=double  SaturateOnIntegerOverflow=on
  Data Type Conversion8 : DataTypeConversion  OutDataTypeStr=boolean  SaturateOnIntegerOverflow=on
  Data Type Conversion9 : DataTypeConversion  OutDataTypeStr=double  SaturateOnIntegerOverflow=on
  CVW_0B : Outport
  wires:
  Data Type Conversion1/1 -> Bus Creator3/1  "SPN1760_GrossCombinationVehicleWeight"
  CVW_0B1/1 -> Data Type Conversion1/1
  Data Type Conversion9/1 -> Bus Creator3/3  "RX_time"
  Data Type Conversion10/1 -> Bus Creator3/4  "RX_delta_time"
  Data Type Conversion8/1 -> Bus Creator3/2  "RX_status"
  CVW_0B1/2 -> Data Type Conversion8/1
  CVW_0B1/3 -> Data Type Conversion9/1
  CVW_0B1/4 -> Data Type Conversion10/1
  Enable/1 -> CVW_0B1/Enable
  Bus Creator3/1 -> CVW_0B/1  "CVW_0B"
